simulink model "jian4xie2zhen4zi3"  (Simulink 5.0)
settings: Solver=ode45  StartTime=0.0  StopTime=50  RelTol=1e-10
libraries: simulink x1
settings Model: LastModifiedBy=Administrator

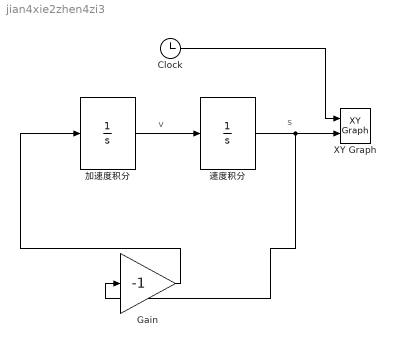
== system jian4xie2zhen4zi3 ==
  note: v
  note: s
  Clock : Clock
      settings: Decimation=10
  Gain : Gain  Gain=-1  SaturateOnIntegerOverflow=on
  XY Graph : simulink/Sinks/XY Graph  xmin=-1  xmax=50  ymin=-8  ymax=8  st=-1
  加速度积分 : Integrator
  速度积分 : Integrator  InitialCondition=1
  wires:
  加速度积分/1 -> 速度积分/1
  速度积分/1 -> XY Graph/2, Gain/1
  Gain/1 -> 加速度积分/1
  Clock/1 -> XY Graph/1
